simulink model "Control5_SF_pose2vw"  (R2023b)
settings: Solver=FixedStepAuto  StartTime=0.0  StopTime=40  RelTol=1e-3  EnableMultiTasking=on
model workspace (MAT data in the model file):
  d = 0.15
settings Model: ExtModeTrigDuration=2  Creator=Usuario  LastModifiedBy=Usuario
settings OptimizationCC: EnhancedBackFolding=on  PassReuseOutputArgsAs=Individual arguments  ZeroExternalMemoryAtStartup=off  ZeroInternalMemoryAtStartup=off  MaxStackSize=64  OptimizeBlockOrder=speed  DifferentSizesBufferReuse=on  OptimizationCustomize=off  EfficientTunableParamExpr=on
settings DebuggingCC: ParameterTunabilityLossMsg=error
settings HardwareCC: ProdBitPerInt=16  ProdBitPerPointer=16  ProdBitPerSizeT=16  ProdBitPerPtrDiffT=16  ProdLargestAtomicFloat=None  ProdWordSize=8  ProdHWDeviceType=Atmel->AVR  UseEmbeddedCoderFeatures=off  UseSimulinkCoderFeatures=off
settings SFSimCC: MATLABDynamicMemAlloc=off
settings RTWCC: Description=Embedded Coder  SystemTargetFile=ert.tlc  HardwareBoard=Arduino Mega 2560  TemplateMakefile=ert_default_tmf  Toolchain=Arduino AVR  BuildConfiguration=Faster Runs
settings CodeAppCC: ForceParamTrailComments=on  IgnoreCustomStorageClasses=off  OperatorAnnotations=on  SimulinkDataObjDesc=on  SFDataObjDesc=on  InsertBlockDesc=on
settings ERTTargetCC: SupportContinuousTime=on  SupportNonInlinedSFcns=on  SupportVariableSizeSignals=on  ExtModeTransport=3  ExtModeStaticAlloc=on  ExtModeAutomaticAllocSize=off  ExtModeStaticAllocSize=2048  ExtModeMexFile=ext_xcp  ExtModeIntrfLevel=Level2 - Open

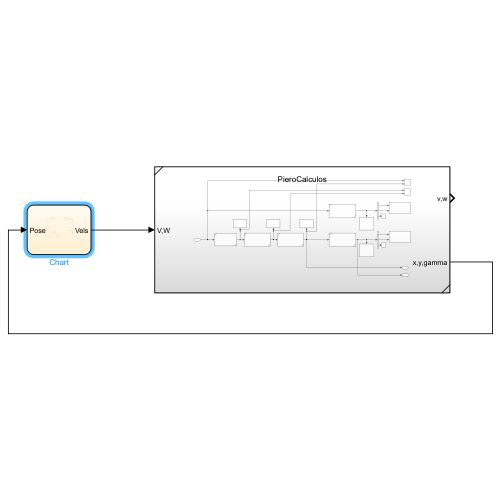
[thumbnail: Simulink's stored preview of the top-level diagram]
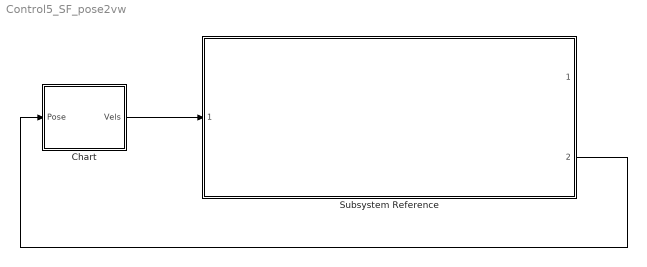
== system Control5_SF_pose2vw ==
  Chart : Stateflow chart  TreatAsAtomicUnit=on
  Subsystem Reference : Subsystem  ReferencedSubsystem=PieroCalculos
  wires:
  Chart/1(Vels) -> Subsystem Reference/1
  Subsystem Reference/2 -> Chart/1(Pose)

== stateflow chart Control5_SF_pose2vw/Chart ==
  state Avanza3
    entry:
    Vels(1)=0.25;
    Vels(2)=0;
  state Giro2
    entry:
    Vels(1)=0;
    Vels(2)=-pi/2;
  state Giro1
    entry:
    Vels(1)=0;
    Vels(2)=-pi/2;
  state Avanza4
    entry:
    Vels(1)=0.25;
    Vels(2)=0;
  state Avanza2
    entry:
    Vels(1)=0.25;
    Vels(2)=0;
  state Giro3
    entry:
    Vels(1)=0;
    Vels(2)=pi/2;
  state Circunferencia
    entry:
    Vels(1)=0.25;
    Vels(2)=-pi/10;
  state Avanza5
    entry:
    Vels(1)=0.25;
    Vels(2)=0;
  state Inicio
    entry:
    Vels(1)=0;
    Vels(2)=0;
  state Avanza1
    entry:
    Vels(1)=0.25;
    Vels(2)=0;
  state Giro_180
    entry:
    Vels(1)=0;
    Vels(2)=-pi/2;
  state Parada
    entry:
    Vels(1)=0;
    Vels(2)=0;
  Giro2 -> Avanza4 : [Pose(3)<=-5*pi/2]
  Giro1 -> Avanza3 : [Pose(3)<=-2*pi]
  Avanza3 -> Giro2 : [Pose(1)>=1.9]
  Avanza2 -> Giro1 : [Pose(2)>=1.6]
  Avanza4 -> Giro3 : [Pose(2)<=0]
  Circunferencia -> Avanza2 : [Pose(3)<=-3*pi/2]
  Giro_180 -> Circunferencia : [Pose(3)<=-pi]
  (default) -> Inicio
  Giro3 -> Avanza5 : [Pose(3)>=-9*pi/4]
  Inicio -> Avanza1 : [after(1,sec)]
  Avanza5 -> Parada : [Pose(1)>=1.9+cos(-pi/4) || Pose(2)<=sin(-pi/4)]
  Avanza1 -> Giro_180 : [Pose(1)>=1.15]
  data: Vels output double size=2; Pose input double size=3
